simulink model "statefdbk"  (Simulink 8.5)
settings: Solver=ode45  StartTime=0.0  StopTime=T  RelTol=1e-3
values from neighbouring files (symbols this model uses):
  C = eye(5,5)    [Home.m]
  D = zeros(1,2)    [Home.m]    (also in analysis.m)
  K = lqr(A, B, Qr, Rr)    [Home.m]    (also in analysis.m; fp_ini.m)
  x0 = [alpha 0 beta 0 0]'    [Home.m]    (also in analysis.m)
undefined symbols (not defined in the file or in its folder): A, B
settings Model: Creator=João Pedro Belfo  LastModifiedBy=luisr
settings DataIOCC: SignalLoggingSaveFormat=Dataset
settings OptimizationCC: ExpressionDepthLimit=128
settings DebuggingCC: UnderspecifiedInitializationDetection=Simplified  MergeDetectMultiDrivingBlocksExec=error  FcnCallInpInsideContextMsg=EnableAllAsError  StateNameClashWarn=none
settings GRTTargetCC: CombineOutputUpdateFcns=on  GRTInterface=off

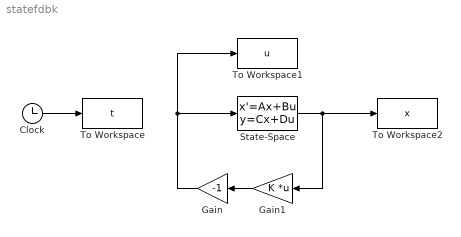
== system statefdbk ==
  Clock : Clock
  Gain : Gain  Gain=-1
  Gain1 : Gain  Gain=K  Multiplication=Matrix(K*u)
  State-Space : StateSpace  A=A  B=B  C=C  D=D  X0=x0
  To Workspace : ToWorkspace  VariableName=t  SaveFormat=Timeseries  SampleTime=-1
  To Workspace1 : ToWorkspace  VariableName=u  SaveFormat=Timeseries  SampleTime=-1
  To Workspace2 : ToWorkspace  VariableName=x  SaveFormat=Timeseries  SampleTime=-1
  wires:
  Clock/1 -> To Workspace/1
  Gain1/1 -> Gain/1
  State-Space/1 -> Gain1/1, To Workspace2/1
  Gain/1 -> To Workspace1/1, State-Space/1
